simulink model "slexFMCWMultiTargetsExample"  (R2018b)
settings: Solver=FixedStepDiscrete  StartTime=0.0  StopTime=2*64*paramFMCWMT.T  RelTol=1e-3  EnableMultiTasking=on
PreLoadFcn:
  | helperslexFMCWMultiTargetsParam
undefined symbols (not defined in the file or in its folder): paramFMCWMT, parula
libraries: phasedenvlib x7, phasedtxrxlib x2, phaseddetectlib x2, phasedwavlib x1, dspmathops x1
CloseFcn:
  | clear paramFMCWMT
Description:
  | FMCW Radar Range Estimation
  | 
  | This model shows how to use a FMCW radar to estimate a target's range.
settings Model: Creator=The MathWorks, Inc.  LastModifiedBy=The MathWorks, Inc.
settings DataIOCC: LimitDataPoints=on  SaveFormat=Array
settings OptimizationCC: LifeSpan=inf
settings DebuggingCC: ReadBeforeWriteMsg=DisableAll  WriteAfterWriteMsg=DisableAll  WriteAfterReadMsg=DisableAll  UnderspecifiedInitializationDetection=Classic  MergeDetectMultiDrivingBlocksExec=none  SolverPrmCheckMsg=warning  MultiTaskDSMMsg=none  LibraryContextMissingDiagnostic=none  SFUnexpectedBacktrackingDiag=warning  SFNoUnconditionalDefaultTransitionDiag=warning  SFExecutionAtInitializationDiag=none
settings HardwareCC: ProdBitPerPointer=32  ProdBitPerSizeT=32  ProdBitPerPtrDiffT=32  ProdLargestAtomicFloat=None  ProdIntDivRoundTo=Undefined  ProdEndianess=Unspecified  ProdWordSize=32  ProdHWDeviceType=32-bit Generic
settings ModelReferenceCC: UpdateModelReferenceTargets=IfOutOfDate  PropagateSignalLabelsOutOfModel=off
settings SFSimCC: SFSimEcho=off  SimUseLocalCustomCode=off
settings RTWCC: RTWUseLocalCustomCode=off
settings CodeAppCC: StateflowObjectComments=on
settings GRTTargetCC: TargetLangStandard=C89/C90 (ANSI)  GeneratePreprocessorConditionals=Disable all
settings ConfigComp: CovMetricSettings=dw  CovHtmlReporting=on  CovSaveCumulativeToWorkspaceVar=on  CovSaveSingleToWorkspaceVar=on  CovExternalEMLEnable=off  CovSFcnEnable=off

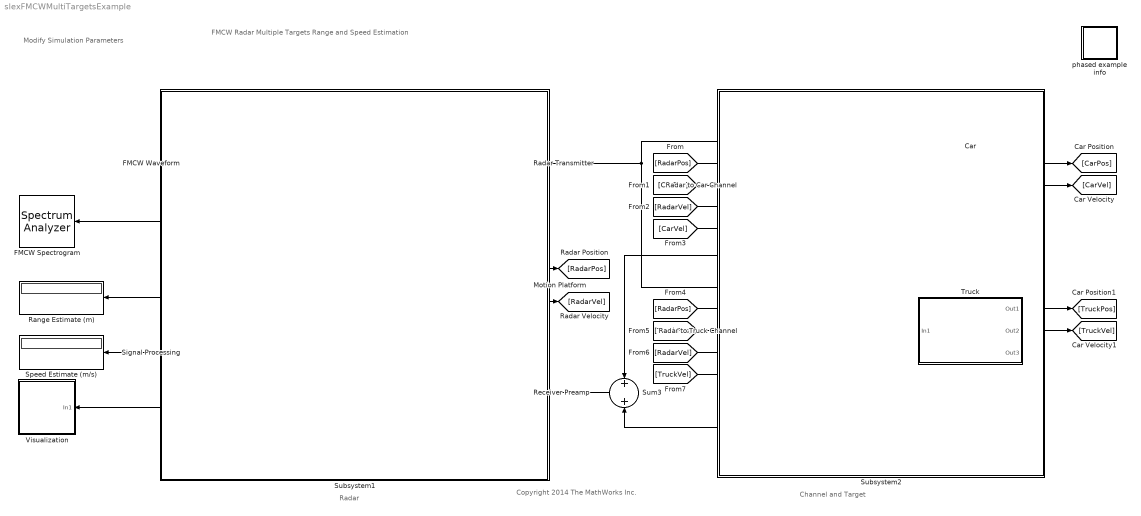
== system slexFMCWMultiTargetsExample ==
  note: Copyright 2014 The MathWorks Inc.
  note: Radar
  note: Channel and Target
  note: FMCW Radar Multiple Targets Range and Speed Estimation
  note: Modify Simulation Parameters
  Car : Subsystem
      mask Display:
      | disp('Car')
      | port_label('output',1,'Pos')
      | port_label('output',2,'Vel')
      | port_label('output',3,'Sig')
  FMCW Spectrogram : SpectrumAnalyzer
  FMCW Waveform : phasedwavlib/FMCW Waveform  SampleRate=paramFMCWMT.Fs  SweepTime=paramFMCWMT.T  SweepBandwidth=paramFMCWMT.bw  SweepDirection=Up  SweepInterval=Symmetric  OutputFormat=Sweeps  NumSamples=100  NumSweeps=1  SimulateUsing=Interpreted execution
      settings: SourceProductName=Phased Array System Toolbox  SourceProductBaseCode=AR
  Motion Platform : phasedenvlib/Motion Platform  MotionModel=Velocity  InitialPosition=paramFMCWMT.RadarPos  InitialVelocity=[ 0; 0; 0 ]  VelocitySource=Property  Velocity=paramFMCWMT.RadarVel  AccelerationSource=Property  Acceleration=[0;0;0]  CustomTrajectory=[ 0, 0, 0, 0, 0, 0, 0; 1, 0, 0, 0, 0, 0, 0 ]  ScanMode=None  InitialScanAngle=0  AzimuthSpan=[ -60, 60 ]  AzimuthScanRate=10  InitialOrientationAxes=eye( 3 )  OrientationAxesOutputPort=off  ElapsedTimeSource=Auto  SampleRateFromInputCheckbox=on  SampleRate=1e6  SimulateUsing=Interpreted execution
      settings: SourceProductName=Phased Array System Toolbox  SourceProductBaseCode=AR
  Radar Transmitter : phasedtxrxlib/Transmitter  PeakPower=paramFMCWMT.ppow  Gain=paramFMCWMT.TxGain  LossFactor=0  InUseOutputPort=off  CoherentOnTransmit=on  PhaseNoiseOutputPort=off  SeedSource=Auto  Seed=0  SimulateUsing=Interpreted execution
      settings: SourceProductName=Phased Array System Toolbox  SourceProductBaseCode=AR
  Radar to Car Channel : phasedenvlib/Free Space  PropagationSpeed=paramFMCWMT.C  OperatingFrequency=paramFMCWMT.Fc  TwoWayPropagation=on  SampleRateFromInputCheckbox=on  SampleRate=1e6  MaximumDistanceSource=Property  MaximumDistance=10e3  MaximumNumInputSamplesSource=Auto  MaximumNumInputSamples=1000  SimulateUsing=Interpreted execution
      settings: SourceProductName=Phased Array System Toolbox  SourceProductBaseCode=AR
  Radar to Truck Channel : phasedenvlib/Free Space  PropagationSpeed=paramFMCWMT.C  OperatingFrequency=paramFMCWMT.Fc  TwoWayPropagation=on  SampleRateFromInputCheckbox=on  SampleRate=1e6  MaximumDistanceSource=Property  MaximumDistance=10e3  MaximumNumInputSamplesSource=Auto  MaximumNumInputSamples=1000  SimulateUsing=Interpreted execution
      settings: SourceProductName=Phased Array System Toolbox  SourceProductBaseCode=AR
  Range Estimate (m) : Display
  Receiver Preamp : phasedtxrxlib/Receiver Preamp  Gain=paramFMCWMT.RxGain  LossFactor=0  NoiseMethod=Noise temperature  NoiseFigure=paramFMCWMT.NF  ReferenceTemperature=290  SampleRateFromInputCheckbox=on  SampleRate=1e6  NoisePower=0  EnableInputPort=off  PhaseNoiseInputPort=off  SeedSource=Auto  Seed=0  SimulateUsing=Interpreted execution
      settings: SourceProductName=Phased Array System Toolbox  SourceProductBaseCode=AR
  Signal Processing : Subsystem
      mask Display:
      | disp('Signal\nProcessing')
      | port_label('input',1,'Ref')
      | port_label('input',2,'Echo')
      | port_label('output',1,'Range')
      | port_label('output',2,'Speed')
      | port_label('output',3,'RD')
  Speed Estimate (m/s) : Display
  Subsystem1 : Subsystem
  Subsystem2 : Subsystem
  Sum3 : Sum  Inputs=+|+
  Truck : Subsystem
      mask Display:
      | disp('Truck')
      | port_label('output',1,'Pos')
      | port_label('output',2,'Vel')
      | port_label('output',3,'Sig')
  Visualization : Subsystem
      mask Display: disp('Range-Doppler\nVisualization')
  phased example info : Subsystem
      settings: OpenFcn=|
      | modelname = 'slexFMCWExample';
      | helpview(fullfile(matlabroot,'help','phased','helptargets.map'),sprintf('%sExample',modelname));
      | clear modelname;
      mask Display: disp('Info')
  wires:
  FMCW Waveform/1 -> Signal Processing/1(In1), FMCW Spectrogram/1, Radar Transmitter/1
  [RadarPos] -> Radar to Car Channel/2
  [CarPos] -> Radar to Car Channel/3
  [RadarVel] -> Radar to Car Channel/4
  [CarVel] -> Radar to Car Channel/5
  Radar Transmitter/1 -> Radar to Truck Channel/1, Radar to Car Channel/1
  Motion Platform/1 -> [RadarPos]
  Motion Platform/2 -> [RadarVel]
  Radar to Car Channel/1 -> Car/1(In1)
  Car/1(Out1) -> [CarPos]
  Car/2(Out2) -> [CarVel]
  Truck/1(Out1) -> [TruckPos]
  Truck/2(Out2) -> [TruckVel]
  Radar to Truck Channel/1 -> Truck/1(In1)
  [RadarPos] -> Radar to Truck Channel/2
  [TruckPos] -> Radar to Truck Channel/3
  [RadarVel] -> Radar to Truck Channel/4
  [TruckVel] -> Radar to Truck Channel/5
  Car/3(Out3) -> Sum3/1
  Sum3/1 -> Receiver Preamp/1
  Truck/3(Out3) -> Sum3/2
  Receiver Preamp/1 -> Signal Processing/2(In2)
  Signal Processing/1(Out1) -> Range Estimate (m)/1
  Signal Processing/2(Out2) -> Speed Estimate (m/s)/1
  Signal Processing/3(Out3) -> Visualization/1(In1)

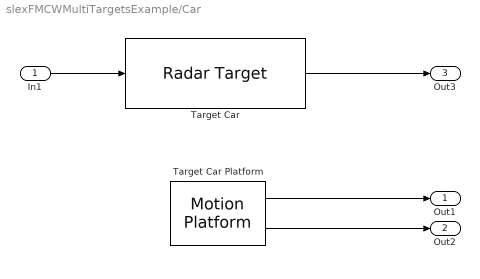
== system slexFMCWMultiTargetsExample/Car ==
  In1 : Inport
  Target Car : phasedenvlib/Radar Target  EnablePolarization=off  Mode=Monostatic  MeanRCSSource=Property  ScatteringMatrixSource=Property  MeanRCS=paramFMCWMT.RCS  ScatteringMatrix=eye( 2 )  Model=Nonfluctuating  PropagationSpeed=paramFMCWMT.C  OperatingFrequency=paramFMCWMT.Fc  SeedSource=Auto  Seed=0  SimulateUsing=Interpreted execution
      settings: SourceProductName=Phased Array System Toolbox  SourceProductBaseCode=AR
  Target Car Platform : phasedenvlib/Motion Platform  MotionModel=Velocity  InitialPosition=paramFMCWMT.CarPos  InitialVelocity=[ 0; 0; 0 ]  VelocitySource=Property  Velocity=paramFMCWMT.CarVel  AccelerationSource=Property  Acceleration=[0;0;0]  CustomTrajectory=[ 0, 0, 0, 0, 0, 0, 0; 1, 0, 0, 0, 0, 0, 0 ]  ScanMode=None  InitialScanAngle=0  AzimuthSpan=[ -60, 60 ]  AzimuthScanRate=10  InitialOrientationAxes=eye( 3 )  OrientationAxesOutputPort=off  ElapsedTimeSource=Auto  SampleRateFromInputCheckbox=on  SampleRate=1e6  SimulateUsing=Interpreted execution
      settings: SourceProductName=Phased Array System Toolbox  SourceProductBaseCode=AR
  Out1 : Outport
  Out2 : Outport  Port=2
  Out3 : Outport  Port=3
  wires:
  Target Car/1 -> Out3/1
  In1/1 -> Target Car/1
  Target Car Platform/1 -> Out1/1
  Target Car Platform/2 -> Out2/1

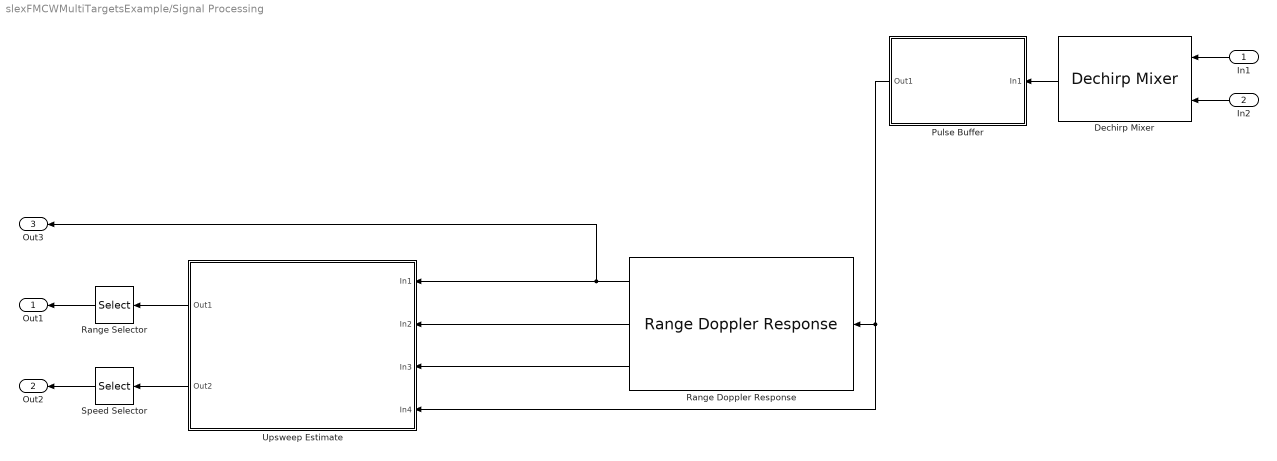
== system slexFMCWMultiTargetsExample/Signal Processing ==
  In1 : Inport
  In2 : Inport  Port=2
  Dechirp Mixer : phaseddetectlib/Dechirp Mixer
      settings: SourceProductName=Phased Array System Toolbox  SourceProductBaseCode=AR
  Pulse Buffer : Subsystem
      mask Display: disp('Pulse Buffer')
  Range Selector : Selector  InputPortWidth=2  IndexOptions=Index vector (dialog)  Indices=[1 2]  OutputSizes=1
  Range Doppler Response : phaseddetectlib/Range Doppler Response  RangeMethod=FFT  PropagationSpeed=paramFMCWMT.C  SampleRateFromInputCheckbox=on  SampleRate=1e6  SweepSlope=paramFMCWMT.slope  DechirpInput=off  RangeFFTLengthSource=Property  RangeFFTLength=paramFMCWMT.NRangeFFT  RangeWindow=Hamming  RangeSidelobeAttenuation=30  CustomRangeWindow=@hamming  ReferenceRangeCentered=off  ReferenceRange=0  MaximumNumInputSamplesSource=Auto  MaximumNumInputSamples=100  PRFSource=Auto  PRF=10e3  DopplerFFTLengthSource=Property  DopplerFFTLength=paramFMCWMT.NDopplerFFT  DopplerWindow=Hamming  DopplerSidelobeAttenuation=30  CustomDopplerWindow=@hamming  DopplerOutput=Speed  OperatingFrequency=paramFMCWMT.Fc  SimulateUsing=Interpreted execution
      settings: SourceProductName=Phased Array System Toolbox  SourceProductBaseCode=AR
  Speed Selector : Selector  InputPortWidth=2  IndexOptions=Index vector (dialog)  Indices=[1 2]  OutputSizes=1
  Upsweep Estimate : Subsystem
      mask Display:
      | disp('Up Sweep\nRange Speed\nEstimation')
      | 
      | port_label('input',1,'RD')
      | port_label('input',2,'RGrid')
      | port_label('input',3,'VGrid')
      | port_label('input',4,'X')
      | port_label('output',1,'Range')
      | port_label('output',2,'Speed')
  Out1 : Outport
  Out2 : Outport  Port=2
  Out3 : Outport  Port=3
  wires:
  Dechirp Mixer/1 -> Pulse Buffer/1(In1)
  In2/1 -> Dechirp Mixer/2
  Range Doppler Response/1 -> Out3/1, Upsweep Estimate/1(In1)
  Pulse Buffer/1(Out1) -> Upsweep Estimate/4(In4), Range Doppler Response/1
  Range Selector/1 -> Out1/1
  Speed Selector/1 -> Out2/1
  In1/1 -> Dechirp Mixer/1
  Upsweep Estimate/1(Out1) -> Range Selector/1
  Upsweep Estimate/2(Out2) -> Speed Selector/1
  Range Doppler Response/2 -> Upsweep Estimate/2(In2)
  Range Doppler Response/3 -> Upsweep Estimate/3(In3)

== system slexFMCWMultiTargetsExample/Subsystem1 ==

== system slexFMCWMultiTargetsExample/Subsystem2 ==

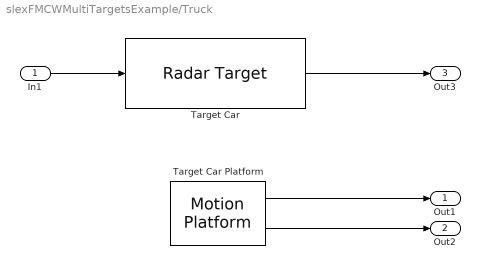
== system slexFMCWMultiTargetsExample/Truck ==
  In1 : Inport
  Target Car : phasedenvlib/Radar Target  EnablePolarization=off  Mode=Monostatic  MeanRCSSource=Property  ScatteringMatrixSource=Property  MeanRCS=paramFMCWMT.TruckRCS  ScatteringMatrix=eye( 2 )  Model=Nonfluctuating  PropagationSpeed=paramFMCWMT.C  OperatingFrequency=paramFMCWMT.Fc  SeedSource=Auto  Seed=0  SimulateUsing=Interpreted execution
      settings: SourceProductName=Phased Array System Toolbox  SourceProductBaseCode=AR
  Target Car Platform : phasedenvlib/Motion Platform  MotionModel=Velocity  InitialPosition=paramFMCWMT.TruckPos  InitialVelocity=[ 0; 0; 0 ]  VelocitySource=Property  Velocity=paramFMCWMT.TruckVel  AccelerationSource=Property  Acceleration=[0;0;0]  CustomTrajectory=[ 0, 0, 0, 0, 0, 0, 0; 1, 0, 0, 0, 0, 0, 0 ]  ScanMode=None  InitialScanAngle=0  AzimuthSpan=[ -60, 60 ]  AzimuthScanRate=10  InitialOrientationAxes=eye( 3 )  OrientationAxesOutputPort=off  ElapsedTimeSource=Auto  SampleRateFromInputCheckbox=on  SampleRate=1e6  SimulateUsing=Interpreted execution
      settings: SourceProductName=Phased Array System Toolbox  SourceProductBaseCode=AR
  Out1 : Outport
  Out2 : Outport  Port=2
  Out3 : Outport  Port=3
  wires:
  Target Car Platform/2 -> Out2/1
  Target Car Platform/1 -> Out1/1
  In1/1 -> Target Car/1
  Target Car/1 -> Out3/1

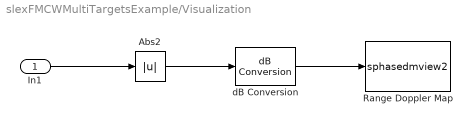
== system slexFMCWMultiTargetsExample/Visualization ==
  In1 : Inport
  Abs2 : Abs
  Range Doppler Map : M-S-Function  DialogController=phaseddialog.MatrixViewer  FunctionName=sphasedmview2  Parameters={CMapStr},YMin,YMax,DataLimits,XData,YData,AxisColorbar,AxisOrigin,{XLabel},{YLabel},{ZLabel},FigPos,AxisZoom  DisplayMFileStacktrace=off  mask(Matrix Viewer){ShowPortLabels=off, ImageParams=off, CMapStr=parula(256), YMin=-127.5752, YMax=4.4686, DataLimits=User-defined, XData=[-131.7841 132.8217]*18/5, YData=[0 1099.4629], AxisColorbar=on, AxisParams=off, AxisOrigin=Upper left corner, XLabel=Speed (km/h), YLabel=Range (m), ZLabel=Power (dB), FigPos=[1271 257 560 420], AxisZoom=off}
      mask prompts: ShowPortLabels "dummy"; ImageParams "-------------------------------- Show Image properties ------------------------------------"; CMapStr "Colormap matrix:"; YMin "Minimum input value:"; YMax "Maximum input value:"; DataLimits "Data limits"; XData "X-Data value:"; YData "Y-Data value:"; AxisColorbar "Display colorbar"; AxisParams "-------------------------------- Show axis properties ----------------------------------------"; AxisOrigin "Axis origin:"; XLabel "X-axis title:"; YLabel "Y-axis title:"; ZLabel "Colorbar title:"; FigPos "Figure position:"; AxisZoom "Axis zoom"
      mask help: Display a matrix as an image, scaling the colormap to the specified input data range. Colormap must be an Nx3 matrix of RGB values. Type "help graph3d" at the MATLAB prompt for a list of predefined colormaps.
      settings: CopyFcn=sphasedmview2([],[],[],'BlockCopy');  DeleteFcn=sphasedmview2([],[],[],'BlockDelete');  NameChangeFcn=sphasedmview2([],[],[],'BlockNameChange');
      mask Help: eval('blocksethelp');
      mask TypeOptions DataLimits: Auto | User-defined
      mask TypeOptions AxisOrigin: Upper left corner | Lower left corner
      mask Display: disp('Range Doppler\nViewer')
  dB Conversion : dspmathops/dB Conversion  dBtype=dB  intype=Amplitude  R=1  fuzz=on
      settings: SourceProductName=DSP System Toolbox
  wires:
  In1/1 -> Abs2/1
  dB Conversion/1 -> Range Doppler Map/1
  Abs2/1 -> dB Conversion/1

== system slexFMCWMultiTargetsExample/phased example info ==

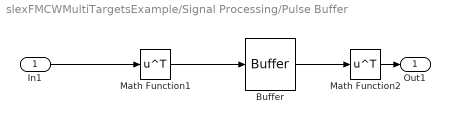
== system slexFMCWMultiTargetsExample/Signal Processing/Pulse Buffer ==
  In1 : Inport
  Buffer : Buffer  N=paramFMCWMT.NBuffer  V=paramFMCWMT.NBuffer-1
  Math Function1 : Math  Operator=transpose  OutputSignalType=complex  SaturateOnIntegerOverflow=on
  Math Function2 : Math  Operator=transpose  OutputSignalType=complex  SaturateOnIntegerOverflow=on
  Out1 : Outport
  wires:
  Buffer/1 -> Math Function2/1
  In1/1 -> Math Function1/1
  Math Function2/1 -> Out1/1
  Math Function1/1 -> Buffer/1

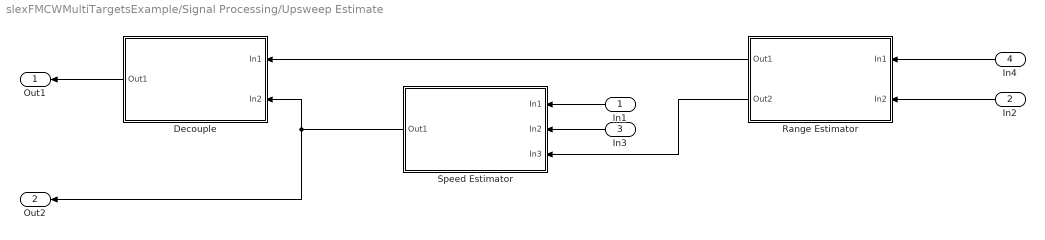
== system slexFMCWMultiTargetsExample/Signal Processing/Upsweep Estimate ==
  In1 : Inport
  In2 : Inport  Port=2
  In3 : Inport  Port=3
  In4 : Inport  Port=4
  Decouple : Subsystem
      mask Display:
      | disp('Range Doppler\nDecoupler')
      | port_label('input',1,'Range')
      | port_label('input',2,'Speed')
      | port_label('output',1,'Range')
  Range Estimator : Subsystem
      mask Display:
      | disp('Range\nEstimator')
      | port_label('input',1,'X')
      | port_label('input',2,'RGrid')
      | port_label('output',1,'Range')
      | port_label('output',2,'Idx')
  Speed Estimator : Subsystem
      mask Display:
      | disp('Speed\nEstimator')
      | port_label('input',1,'RD')
      | port_label('input',2,'SGrid')
      | port_label('input',3,'Idx')
      | port_label('output',1,'Speed')
  Out1 : Outport
  Out2 : Outport  Port=2
  wires:
  In4/1 -> Range Estimator/1(In1)
  In2/1 -> Range Estimator/2(In2)
  Speed Estimator/1(Out1) -> Out2/1, Decouple/2(In2)
  Range Estimator/2(Out2) -> Speed Estimator/3(In3)
  In3/1 -> Speed Estimator/2(In2)
  In1/1 -> Speed Estimator/1(In1)
  Range Estimator/1(Out1) -> Decouple/1(In1)
  Decouple/1(Out1) -> Out1/1

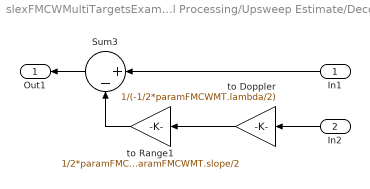
== system slexFMCWMultiTargetsExample/Signal Processing/Upsweep Estimate/Decouple ==
  In1 : Inport
  In2 : Inport  Port=2
  Sum3 : Sum  Inputs=|+-
  to Doppler : Gain  Gain=1/(-1/2*paramFMCWMT.lambda/2)
  to Range1 : Gain  Gain=1/2*paramFMCWMT.C/paramFMCWMT.slope/2
  Out1 : Outport
  wires:
  to Doppler/1 -> to Range1/1
  In2/1 -> to Doppler/1
  Sum3/1 -> Out1/1
  to Range1/1 -> Sum3/2
  In1/1 -> Sum3/1

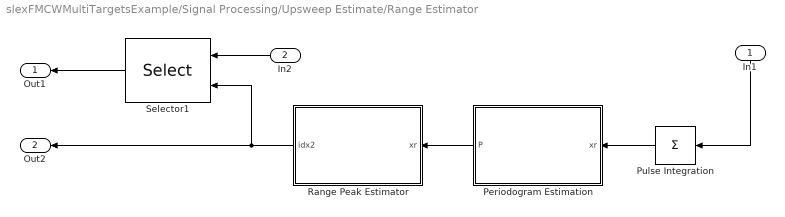
== system slexFMCWMultiTargetsExample/Signal Processing/Upsweep Estimate/Range Estimator ==
  In1 : Inport
  In2 : Inport  Port=2
  Periodogram Estimation : MATLAB Function  TreatAsAtomicUnit=on  mask(Periodogram Estimation){N=paramFMCWMT.NRangeFFT}
      mask prompts: N "Number of FFT Points"
      mask help: Compute Periodogram
  Pulse Integration : Sum  Inputs=+  CollapseMode=Specified dimension  CollapseDim=2
  Range Peak Estimator : MATLAB Function  TreatAsAtomicUnit=on
  Selector1 : Selector  InputPortWidth=paramFMCWMT.NRangeFFT  IndexOptions=Index vector (port)  Indices=[1 3]  OutputSizes=1
  Out1 : Outport
  Out2 : Outport  Port=2
  wires:
  In2/1 -> Selector1/1
  Periodogram Estimation/1(P) -> Range Peak Estimator/1(xr)
  Pulse Integration/1 -> Periodogram Estimation/1(xr)
  Range Peak Estimator/1(idx2) -> Selector1/2, Out2/1
  Selector1/1 -> Out1/1
  In1/1 -> Pulse Integration/1

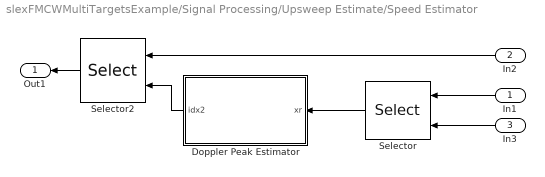
== system slexFMCWMultiTargetsExample/Signal Processing/Upsweep Estimate/Speed Estimator ==
  In1 : Inport
  In2 : Inport  Port=2
  In3 : Inport  Port=3
  Doppler Peak Estimator : MATLAB Function  TreatAsAtomicUnit=on
  Selector : Selector  NumberOfDimensions=2  InputPortWidth=3  IndexOptions=Index vector (port),Select all  Indices=[1 3],1  OutputSizes=1,1
  Selector2 : Selector  InputPortWidth=paramFMCWMT.NDopplerFFT  IndexOptions=Index vector (port)  Indices=[1 3]  OutputSizes=1
  Out1 : Outport
  wires:
  In3/1 -> Selector/2
  Selector2/1 -> Out1/1
  In2/1 -> Selector2/1
  Selector/1 -> Doppler Peak Estimator/1(xr)
  Doppler Peak Estimator/1(idx2) -> Selector2/2
  In1/1 -> Selector/1

== matlab function slexFMCWMultiTargetsExample/Signal Processing/Upsweep Estimate/Range Estimator/Range Peak Estimator ==
  data: xr input; idx2 output
function idx2 = fcn(xr)
%#codegen

[dummy,idx] = findpeaks(abs(xr(:).'),'NPeaks',2,'SortStr','descend',...
    'MinPeakDistance',100); %#ok<ASGLU>
if ~isempty(idx)
    idx2 = idx(1:2);
else
    idx2 = [floor(numel(xr)/2)+1 floor(numel(xr)/2)+1];
end

== matlab function slexFMCWMultiTargetsExample/Signal Processing/Upsweep Estimate/Speed Estimator/Doppler Peak Estimator ==
  data: xr input; idx2 output
function idx2 = fcn(xr)
%#codegen

idx2 = ones(1,2);
for m = 1:2
    [dummy,idx] = findpeaks(abs(xr(m,:).'),'NPeaks',1,'SortStr','descend'); %#ok<ASGLU>
    if ~isempty(idx)
        idx2(m) = idx(1);
    else
        idx2(m) = floor(size(xr,1)/2)+1;
    end
end

== matlab function slexFMCWMultiTargetsExample/Signal Processing/Upsweep Estimate/Range Estimator/Periodogram Estimation ==
  data: xr input; P output; N parameter
function P = fcn(xr,N)
%#codegen

P = abs(fft(xr(:),N)).^2;
